simulink model "g_closed_loop_speed_simulation"  (R2025a)
settings: Solver=VariableStepAuto  StartTime=0.0  StopTime=1.5  RelTol=1e-3
values from neighbouring files (symbols this model uses):
  B = 0    [Simulink_support_script.m]    (also in quick_pole_check.m)
  Jm = 5.508e-5    (= 5.508e-05)    [Simulink_support_script.m]
  K = 0.0991    [HW2_pro1_min_ab_plot_script.m]    (also in Simulink_support_script.m; quick_pole_check.m)
  Kia = 2*pi*10*Kpa    (= 281.875901695)    [Simulink_support_script.m]
  Kiw = Jm*(2*pi*40)^2    (= 3.47915398664)    [Simulink_support_script.m]
  Kpa = 2*pi*300*L    (= 4.48619430933)    [Simulink_support_script.m]
  Kpw = Jm*2*(2*pi*40)    (= 0.0276862277376)    [Simulink_support_script.m]
  L = 2.38e-3    (= 0.00238)    [Simulink_support_script.m]    (also in quick_pole_check.m = max(xr, yr))
  R = 1.43    [Simulink_support_script.m]    (also in quick_pole_check.m)
  stim_step = 100    [Simulink_support_script.m]
  Tl_final = 0.5    [Simulink_support_script.m]
  Tl_initial = 0    [Simulink_support_script.m]
  Tl_step_t = 0.05    [Simulink_support_script.m]
settings Model: Creator=lpurd  LastModifiedBy=lpurd

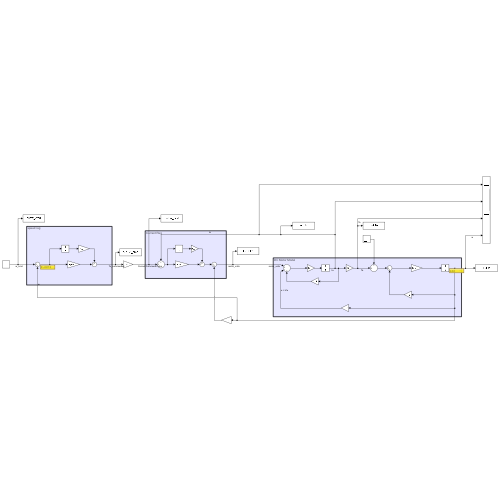
[thumbnail: Simulink's stored preview of the top-level diagram]
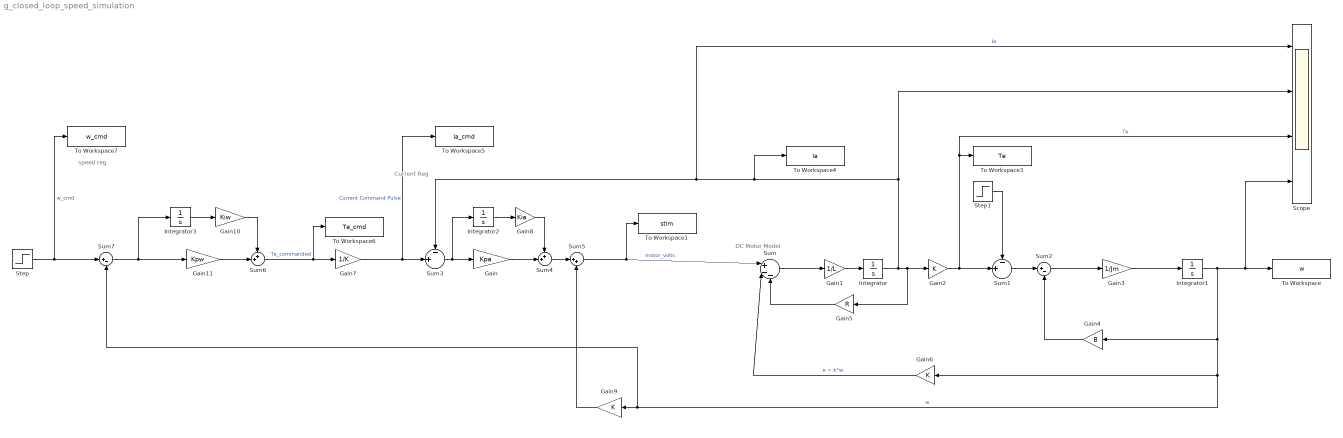
== system g_closed_loop_speed_simulation ==
  note: speed reg
  note: Current Reg
  note: DC Motor Model
  Gain : Gain  Gain=Kpa
  Gain1 : Gain  Gain=1/L
  Gain10 : Gain  Gain=Kiw
  Gain11 : Gain  Gain=Kpw
  Gain2 : Gain  Gain=K
  Gain3 : Gain  Gain=1/Jm
  Gain4 : Gain  Gain=B
  Gain5 : Gain  Gain=R
  Gain6 : Gain  Gain=K
  Gain7 : Gain  Gain=1/K
  Gain8 : Gain  Gain=Kia
  Gain9 : Gain  Gain=K
  Integrator{,1..3} (4 alike) : Integrator
  Scope : Scope  NumInputPorts=4
      settings: ActiveDisplayYMinimum=-1.6047476575996962  ActiveDisplayYMaximum=12.932594199737292
  Step : Step  Time=0  After=stim_step  SampleTime=0
  Step1 : Step  Time=Tl_step_t  Before=Tl_initial  After=Tl_final  SampleTime=0
  Sum : Sum  Inputs=|+--
  Sum1 : Sum  Inputs=-|+||
  Sum2 : Sum  Inputs=|+-
  Sum3 : Sum  Inputs=-|+||
  Sum4 : Sum  Inputs=++|
  Sum5 : Sum  Inputs=|++
  Sum6 : Sum  Inputs=++|
  Sum7 : Sum  Inputs=|+-
  To Workspace : ToWorkspace  VariableName=w  SaveFormat=Timeseries  SampleTime=-1
  To Workspace1 : ToWorkspace  VariableName=stim  SaveFormat=Timeseries  SampleTime=-1
  To Workspace3 : ToWorkspace  VariableName=Te  SaveFormat=Timeseries  SampleTime=-1
  To Workspace4 : ToWorkspace  VariableName=Ia  SaveFormat=Timeseries  SampleTime=-1
  To Workspace5 : ToWorkspace  VariableName=Ia_cmd  SaveFormat=Timeseries  SampleTime=-1
  To Workspace6 : ToWorkspace  VariableName=Te_cmd  SaveFormat=Timeseries  SampleTime=-1
  To Workspace7 : ToWorkspace  VariableName=w_cmd  SaveFormat=Timeseries  SampleTime=-1
  wires:
  Gain6/1 -> Sum/2  "e = k*w"
  Gain4/1 -> Sum2/2
  Gain5/1 -> Sum/3
  Gain2/1 -> To Workspace3/1, Scope/3, Sum1/2  "Te"
  Sum1/1 -> Sum2/1
  Sum2/1 -> Gain3/1
  Step1/1 -> Sum1/1
  Gain3/1 -> Integrator1/1
  Integrator1/1 -> Scope/4, To Workspace/1, Sum7/2, Gain9/1, Gain6/1, Gain4/1  "w"
  Sum/1 -> Gain1/1
  Gain1/1 -> Integrator/1
  Integrator/1 -> Gain5/1, Gain2/1, Scope/2, To Workspace4/1, Scope/1, Sum3/1  "Ia"
  Sum5/1 -> Sum/1, To Workspace1/1  "motor_volts"
  Sum3/1 -> Integrator2/1, Gain/1
  Integrator2/1 -> Gain8/1
  Gain8/1 -> Sum4/1
  Gain/1 -> Sum4/2
  Sum4/1 -> Sum5/1
  Gain9/1 -> Sum5/2
  Gain7/1 -> To Workspace5/1, Sum3/2  "Current Command Pulse"
  Sum6/1 -> To Workspace6/1, Gain7/1  "Te_commanded"
  Integrator3/1 -> Gain10/1
  Gain10/1 -> Sum6/1
  Gain11/1 -> Sum6/2
  Sum7/1 -> Gain11/1, Integrator3/1
  Step/1 -> To Workspace7/1, Sum7/1  "w_cmd"
